simulink model "vehicle_control"  (R2020b)
settings: Solver=VariableStepAuto  StartTime=0.0  StopTime=10.0  RelTol=1e-3
libraries: robotlib x2
settings Model: Creator=safwan  LastModifiedBy=safwan

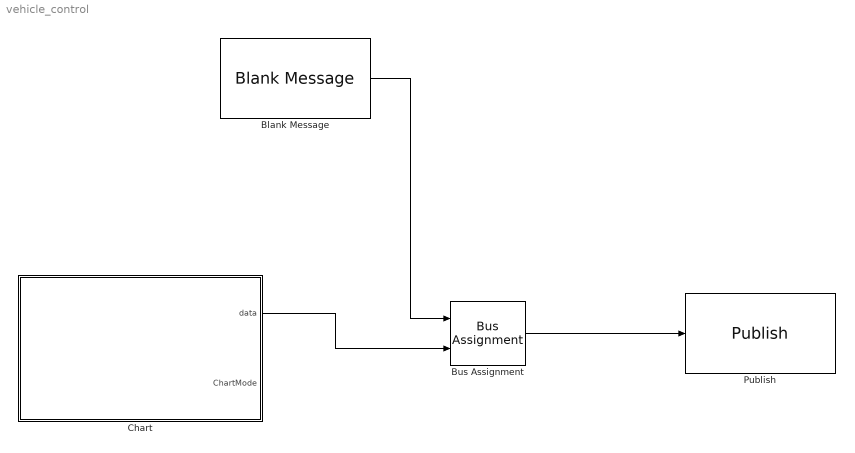
== system vehicle_control ==
  Blank Message : robotlib/Blank Message  messageClass=Message  entityType=std_msgs/Float64  messageType=std_msgs/Float64  SampleTime=-1  legacyBusStruct=off
  Bus Assignment : BusAssignment  AssignedSignals=signal1
  Chart : Stateflow chart  TreatAsAtomicUnit=on
  Publish : robotlib/Publish  topicSource=Specify your own  topic=/commands  messageType=geometry_msgs/Point  legacyBusStruct=off  messageQueueLength=1
  wires:
  Chart/1(data) -> Bus Assignment/2
  Blank Message/1 -> Bus Assignment/1
  Bus Assignment/1 -> Publish/1

== stateflow chart vehicle_control/Chart ==
  state entry_ x = 0.0
  state ?
  state ?
  (default) -> entry_ x = 0.0
  data: data output; ChartMode output Enum: ChartModeType
